simulink model "F16ASYM_Controlled_ACC"  (R2012b)
settings: Solver=ode3  SolverMode=SingleTasking  StartTime=0.0  StopTime=inf  FixedStep=T_sim  RelTol=1e-3
InitFcn:
  | load('NN_c_weights_Last_stable.mat')
values from neighbouring files (symbols this model uses):
  a1 = fitresult.p1    [Stall_protection.m]
  alpha_map_eval = ones(size(M_eval))*NaN    [Auto_trim_aid.m]    (also in Autotrim_maps.mat = [nan nan 0.277598136245 0.119432432992 0.0579479097061 0.027)
  beta_map_eval = ones(size(M_eval))*NaN    [Auto_trim_aid.m]    (also in Autotrim_maps.mat = [nan nan -0.00151549403324 0.00117807579006 -0.0052086799721)
  C_L_0 = fitresult.p2    [Stall_protection.m]
  G_eval = NaN*ones(size(M_sq,2),size(H_sq,2))    [Stall_protection.m]
  H_sq = unique(sort(H_sq))    [Stall_protection.m]
  H_sq_autotrim = min( F_envelope.H_1g):2000:max(F_envelope.H_1g)    [Auto_trim_aid.m]    (also in Autotrim_maps.mat = [0 2000 4000 6000 8000 10000 12000 14000 16000 18000])
  K_b_ACC = params(3)    [Cost_function.m]
  K_b_q = params(4)    [Cost_function.m]
  learning = 20    [Scheduling_desing.m]
  M_sq = unique(sort(M_sq))    [Stall_protection.m]
  M_sq_autotrim = 0:0.1:max(F_envelope.M_1g)    [Auto_trim_aid.m]    (also in Autotrim_maps.mat = [0 0.1 0.2 0.3 0.4 0.5 0.6 0.7 0.8 0.9 1 1.1 ... (21 element)
  Model_used_flag = 1    [Scheduling_desing.m]
  reg_param = 1    [Scheduling_desing.m]
  T_sim = 0.04    [Run_me.m]    (also in Scheduling_desing.m = 0.02)
  tau_ACC = params(1)    [Cost_function.m]
  tau_q = params(2)    [Cost_function.m]
  V_Comp_A_w_z_last = [-0.043311742939 0.0085685727899 -0.0213735657625 0.0330213821126 -0.0306555996667 -0.00573122365227 -0.0106441480787 0.0329440631876 0.0177121952361 -0.0290685435098 -0.0181457235686 -0.0361990502411 ... (1250 elements, 50x25)]    [NN_c_weights_Last_stable.mat]
  V_Comp_last = [-0.0421958473648 0.0184516098779 -0.0436695953504 -0.041154016657 0.00216882652165 -0.0388561228631 0.0327521861474 0.0326079628857 0.0227071838361 -0.0338588476214 0.0161615063846 0.00186003522421 ... (1250 elements, 50x25)]    [NN_c_weights_Last_stable.mat]
  velocity = M_eval(I,J)*a    [Auto_trim_aid.m]    (also in Scheduling_desing.m = M_eval_sche(I,J)*a)
  W_Comp_A_w_z_last = [-0.00689921461652 0.00234704735165 -0.000126421245896 0.00121944724496 6.17702028018e-05 -0.000422762754226 -0.000228913732743 -1.1618795843e-05 7.94007436465e-05 0.000588815786054 2.98617078429e-05 -0.00020420127191 ... (153 elements, 3x51)]    [NN_c_weights_Last_stable.mat]
  W_Comp_last = [-0.00864477030284 0.000183920433695 -0.000300268209456 0.00178165628538 -0.000144806488148 -0.000715209966 -0.000733452792184 5.9552378004e-05 0.000293789747621 0.00184648331608 -0.000150090451416 -0.000741280397229 ... (153 elements, 3x51)]    [NN_c_weights_Last_stable.mat]
undefined symbols (not defined in the file or in its folder): B, DiscIntNeverNeededParam, fi_flag_Simulink, k_B, m_B, sigbuilder_block, Stall_curve, Theta_1_roll_last, Theta_2_roll_last, Theta_3_roll_last, trim_control, trim_state, trim_throttle, V_long_lastA_w_z, V_long_lastAoA, V_roll_last, V_roll_lastMOD, V_yaw_last, W_long_lastA_w_z, W_long_lastAoA, W_roll_last, W_roll_lastMOD, W_yaw_last
libraries: Adaptive_FaultTolerantControl x43, F16_Actuator_Library x14, dspsigops x13, simulink x8, dsparch4 x6, simulink_extras x5, aerolibatmos2 x5, aerolibtransform2 x5, dspmtrx3 x3, qcatlib x2, dspvision x2, dspsnks4 x2
(part 2 of 10)

== system F16ASYM_Controlled_ACC/Cockpit/Joystick ==
  Add1 : Sum
  Add2 : Sum
  Aileron : Selector  InputPortWidth=2  IndexOptions=Index vector (dialog)  Indices=1  OutputSizes=1
  Gain : Gain  Gain=0.01  OutDataTypeStr=double
  Gain{1..2,4,8} (4 alike) : Gain
  Gain3 : Gain  Gain=-1
  Gain5 : Gain  Gain=-10
  Gain6 : Gain  Gain=10  OutDataTypeStr=double
  Gain7 : Gain  Gain=-1
  Integrator Limited2 : Integrator  LimitOutput=on  UpperSaturationLimit=400  LowerSaturationLimit=-400
  Integrator Limited3 : Integrator  LimitOutput=on  UpperSaturationLimit=1  LowerSaturationLimit=-1
  Joystick Input : vrlib/Joystick Input  joyid=1  adjustports=on  forcefeed=off
  Manual Switch : ManualSwitch
  Selector1 : Selector  InputPortWidth=5  IndexOptions=Index vector (dialog)  Indices=1:2  OutputSizes=1
  Selector2 : Selector  InputPortWidth=5  IndexOptions=Index vector (dialog)  Indices=3  OutputSizes=1
  Selector3 : Selector  InputPortWidth=5  IndexOptions=Index vector (dialog)  Indices=4:5  OutputSizes=1
  Selector4 : Selector  InputPortWidth=10  IndexOptions=Index vector (dialog)  Indices=1  OutputSizes=1
  Selector5 : Selector  InputPortWidth=10  IndexOptions=Index vector (dialog)  Indices=4  OutputSizes=1
  Selector6 : Selector  InputPortWidth=10  IndexOptions=Index vector (dialog)  Indices=1  OutputSizes=1
  Selector7 : Selector  InputPortWidth=10  IndexOptions=Index vector (dialog)  Indices=4  OutputSizes=1
  elev : Selector  InputPortWidth=2  IndexOptions=Index vector (dialog)  Indices=2  OutputSizes=1
  speed des : Outport
  Throttle : Outport  Port=2
  Long: Acc : Outport  Port=3
  Roll : Outport  Port=4
  sideslip : Outport  Port=5
  wires:
  Integrator Limited3/1 -> Throttle/1  "Throttle"
  Aileron/1 -> Gain1/1
  Manual Switch/1 -> Aileron/1, elev/1
  Joystick Input/1 -> Selector2/1, Selector3/1, Selector1/1
  Selector1/1 -> Manual Switch/1
  Selector3/1 -> Manual Switch/2
  Selector4/1 -> Gain3/1
  Selector5/1 -> Gain4/1
  Gain3/1 -> Add1/1
  Gain4/1 -> Add1/2
  Add1/1 -> Gain/1
  Gain/1 -> Integrator Limited3/1
  elev/1 -> Gain2/1
  Gain1/1 -> Roll/1
  Selector2/1 -> Gain5/1
  Gain2/1 -> Long: Acc/1
  Gain5/1 -> sideslip/1
  Integrator Limited2/1 -> speed des/1  "Throttle"
  Joystick Input/2 -> Selector5/1, Selector7/1, Selector6/1, Selector4/1
  Selector6/1 -> Gain7/1
  Selector7/1 -> Gain8/1
  Gain7/1 -> Add2/1
  Gain8/1 -> Add2/2
  Add2/1 -> Gain6/1
  Gain6/1 -> Integrator Limited2/1

== system F16ASYM_Controlled_ACC/Cockpit/Signal Builder1 ==
  Demux : Demux  Tag=STV Demux
  FromWs : FromWorkspace  Tag=STV FromWs  VariableName=tuvar  SampleTime=0
      SigBuilderData=|
      | common.afterFinalStr = 'Extrapolate'
      | common.sampleTime = 0
      | dataSet.timeRange = [0 30]
      | dataSet.name = 'Group 1'
      | sbobj.Groups.Name = 'Group 1'
      | sbobj.Groups.Signals(1).Name = 'Signal 1'
      | sbobj.Groups.Signals(1).XData = [0 0.5 0.5 2.5 2.5 30]
      | sbobj.Groups.Signals(1).YData = [0 0 -1 -1 0 0]
      | sbobj.Groups.Signals(2).Name = 'Signal 5'
      | sbobj.Groups.Signals(2).XData = [0 4 4 6 6 30]
      | sbobj.Groups.Signals(2).YData = [0 0 1 1 0 0]
      | sbobj.Groups.Signals(3).Name = 'Signal 6'
      | sbobj.Groups.Signals(3).XData = [0 8 8 10 10 30]
      | sbobj.Groups.Signals(3).YData = [0 0 -0.5 -0.5 0 0]
      | sbobj.Groups.Signals(4).Name = 'Signal 7'
      | sbobj.Groups.Signals(4).XData = [0 12 12 14 14 30]
      | sbobj.Groups.Signals(4).YData = [0 0 0.5 0.5 0 0]
      | sbobj.Groups.TimeRange = [0 30]
  Signal 1 : Outport  Tag=STV Outport
  Signal 5 : Outport  Tag=STV Outport  Port=2
  Signal 6 : Outport  Tag=STV Outport  Port=3
  Signal 7 : Outport  Tag=STV Outport  Port=4
  wires:
  FromWs/1 -> Demux/1
  Demux/1 -> Signal 1/1
  Demux/2 -> Signal 5/1
  Demux/3 -> Signal 6/1
  Demux/4 -> Signal 7/1

== system F16ASYM_Controlled_ACC/Cockpit/Signal Builder2 ==
  Demux : Demux  Tag=STV Demux
  FromWs : FromWorkspace  Tag=STV FromWs  VariableName=tuvar  SampleTime=0
      SigBuilderData=|
      | common.afterFinalStr = 'Extrapolate'
      | common.sampleTime = 0
      | dataSet.timeRange = [0 10]
      | dataSet.name = 'Group 1'
      | sbobj.Groups.Name = 'Group 1'
      | sbobj.Groups.Signals(1).Name = 'Signal 1'
      | sbobj.Groups.Signals(1).XData = [0 5 5 8.02 8.02 10]
      | sbobj.Groups.Signals(1).YData = [0 0 -8.15 -8.15 0.64 0.7]
      | sbobj.Groups.Signals(2).Name = 'Signal 2'
      | sbobj.Groups.Signals(2).XData = [0 10]
      | sbobj.Groups.Signals(2).YData = [0 0]
      | sbobj.Groups.Signals(3).Name = 'Signal 3'
      | sbobj.Groups.Signals(3).XData = [0 10]
      | sbobj.Groups.Signals(3).YData = [0 0]
      | sbobj.Groups.Signals(4).Name = 'Signal 4'
      | sbobj.Groups.Signals(4).XData = [0 10]
      | sbobj.Groups.Signals(4).YData = [0 0]
  Signal 1 : Outport  Tag=STV Outport
  Signal 2 : Outport  Tag=STV Outport  Port=2
  Signal 3 : Outport  Tag=STV Outport  Port=3
  Signal 4 : Outport  Tag=STV Outport  Port=4
  wires:
  FromWs/1 -> Demux/1
  Demux/1 -> Signal 1/1
  Demux/2 -> Signal 2/1
  Demux/3 -> Signal 3/1
  Demux/4 -> Signal 4/1

== matlab function F16ASYM_Controlled_ACC/Primary Controller/P controller + adaptive Isolated NN/On-line (adaptive) multi-layer NNs SIMPL/Roll NN/Roll 1HL NN/Roll NN ==
  data: X_bar input size=[8,1]; v_ad_comp output; e input; P input; B input; Roll_learnign_rate input size=1; Roll_reg_param input size=1; W input size=[1,31]; V input size=[30,8]; v_ad output; Z_norm_unit output; T_sim parameter; W_update output size=[1,31]; V_update output size=[30,8]
function [v_ad_comp,v_ad,Z_norm_unit,W_update,V_update]  = Roll_NN(X_bar,e,P,B,Roll_learnign_rate,Roll_reg_param,W,V,T_sim)

%% Compute prelimiary parametes
zeta= e'*P*B;
s=zeros(30,1);
z=s;
%% Feedforward
z = V*X_bar;
s=sigmoid(V*X_bar);

sigma = [1 ; s ];
% v_ad = W*sigma;

sigma_grad = (sigma.*(ones(size(sigma))-sigma));

%% Compute the gradients or adaptation laws
Gamma_w= Roll_learnign_rate; % W learnign rate
Gamma_v= Roll_learnign_rate; %V learning rate
lambda = Roll_reg_param;

V_dot=zeros(size(V));
W_dot=zeros(size(W'));

W_dot= -Gamma_w*(  (sigma - sigma_grad.*[1;z] ).*zeta  );
W_dot(2:end,1)= W_dot(2:end,1) - Gamma_w*lambda*norm(zeta)*(W(:,2:end))';

M = W'*zeta.*sigma_grad ;
V_dot= -Gamma_v*( M(2:end)*X_bar'  );
V_dot(:,2:end)= V_dot(:,2:end) - Gamma_v*lambda*norm(zeta).*V(:,2:end);


% Other way: Based on notes of Andrew NG
% % % % W_dot=zeros(size(W));
% % % % delta2=W'*zeta.*sigma_grad;
% % % % 
% % % % V_dot = - Gamma_v*( delta2(2:end)*X_bar');
% % % % V_dot(:,2:end)= V_dot(:,2:end) - Gamma_v*lambda*norm(zeta).*V(:,2:end);
% % % % 
% % % % W_dot = - Gamma_w*( zeta*sigma');
% % % % W_dot(:,2:end)= W_dot(:,2:end) - Gamma_w*lambda*norm(zeta)*(W(:,2:end));
% % % % 
% % % % W_dot = W_dot';


%% Adaptation
W_update = W + T_sim*W_dot';
V_update = V + T_sim*V_dot;

%% re-compute v_ad

z = V*X_bar;
s=sigmoid(V*X_bar);

sigma = [1 ; s(:,1) ];
v_ad = W*sigma;

%% Compute v_ad_comp
Z = [ V,zeros(size(V,1),size(W,2));
    zeros(size(W,1),size(V,2)),W];
    
Z_norm = norm(Z,'fro');
Z_max = 2*min(size(W,1),size(W,2) )*min( size(V,1),size(V,2) );
Z_norm_unit = Z_norm;

K_r0= 0;
K_r1= 0;
v_r0 = -K_r0*zeta;
v_r1 = -K_r1*(Z_norm+Z_max)*zeta;
v_ad_comp = v_ad + v_r1 +v_r0;

% % K_r1= 1;
% % v_r1 = - K_r1*(Z_norm+Z_max)*zeta;
% % 
% % v_ad_comp = v_ad + v_r1 ;



end

== matlab function F16ASYM_Controlled_ACC/Anti-windup Calculation/Anti-windup: Reconfigurable/Ang Accel ==
  data: L input; p_dot output; q_dot output; r_dot output; M input; N input; omega_b input
function [p_dot,q_dot,r_dot] = Ang_accel(L,M,N,omega_b)
Jy  = 75673.6;
Jxz = 1331.4; 
Jz  = 85552.1;  
Jx  = 12874.8;
h_E = 216.9;

denom = Jx*Jz - Jxz*Jxz;

% % C1 = ((Jy - Jz)  * Jz  - (Jxz * Jxz))/ Gamma;
% % C2 = ((Jx - Jy + Jz ) * Jxz ) / Gamma;
% % C3 = Jz / Gamma;
% % C4 = Jxz / Gamma;
% % C5 = (Jz - Jx) / Jy;
% % C6 = Jxz / Jy ;
% % C7 = 1 / Jy;
% % C8 = (Jx * (Jx - Jy ) + Jxz * Jxz) / Gamma;
% % C9 = Jx / Gamma;


p_dot =  (Jz*L + Jxz*N - (Jz*(Jz-Jy)+Jxz*Jxz)*omega_b(2)*omega_b(3) + Jxz*(Jx-Jy+Jz)*omega_b(1)*omega_b(2) + Jxz*omega_b(2)*h_E)/denom;

q_dot = (M + (Jz-Jx)*omega_b(1)*omega_b(3) - Jxz*(omega_b(1)*omega_b(1)-omega_b(3)*omega_b(3)) - omega_b(3)*h_E)/Jy;


r_dot = (Jx*N + Jxz*L + (Jx*(Jx-Jy)+Jxz*Jxz)*omega_b(1)*omega_b(2) - Jxz*(Jx-Jy+Jz)*omega_b(2)*omega_b(3) +  Jx*omega_b(2)*h_E)/denom;

== matlab function F16ASYM_Controlled_ACC/Anti-windup Calculation/Anti-windup: NO reconfigurable/Antiwindup calculation ==
  data: Ang_acell_comm input; AWU output; Ang_acell_achieved input; Saturations input; B input; deflections input
function AWU = AWU_calculation(Ang_acell_comm,Ang_acell_achieved,Saturations,B,deflections)
% Computing Saturation limits
sup_limit = [24,24,21,21,29,25,25]-1;
inf_limit = [-24,-24,-21,-21,-29,0,0]+1;

for i=1:7
    Saturations(i) = Saturation_smooth(abs(Saturations(i)),deflections(i),sup_limit(i),inf_limit(i));
end
Sat_B = B*Saturations;
B_max = B*ones(7,1);

AWU=zeros(3,1);

%% Method A
% % psi = 0.01; % % of the effort above the one we consider manouvreability is reduced
% % for i=1:3
% %     if i==1 && sign(deflections(3))== sign(deflections(4)) && abs(Sat_B(i))>psi*abs(B_max(i))
% %         AWU(2) = Ang_acell_comm(2) - Ang_acell_achieved(2); % we have to desaturate longitudinally not laterally
% %     elseif  i==1 && sign(deflections(3))~= sign(deflections(4)) && abs(Sat_B(i))>psi*abs(B_max(i))
% %         AWU(i) = Ang_acell_comm(i) - Ang_acell_achieved(i);
% %     elseif i~=1 && abs(Sat_B(i))>psi*abs(B_max(i))
% %         AWU(i) = Ang_acell_comm(i) - Ang_acell_achieved(i);
% %     end 
% % end

%% Method B
% % % % Long
% % % if Saturations(1)~=0 || Saturations(2)~=0 ||  Saturations(6)~=0 || Saturations(7)~=0 || ((Saturations(3)~=0 || Saturations(4)~=0) && sign(deflections(3))== sign(deflections(4)) ) 
% % %     AWU(2) = Ang_acell_comm(2) - Ang_acell_achieved(2);
% % % end
% % % % Lat-dir
% % % if ((Saturations(3)~=0 || Saturations(4)~=0) && sign(deflections(3)) ~= sign(deflections(4)) )  || Saturations(5)~=0 || Saturations(6)~=0 || Saturations(7)~=0
% % %     AWU(1) = Ang_acell_comm(1) - Ang_acell_achieved(1);
% % %     AWU(3) = Ang_acell_comm(3) - Ang_acell_achieved(3);
% % % 
% % % end



%% Method C
for i=1:3
        AWU(i) = (Ang_acell_comm(i) - Ang_acell_achieved(i))*Sat_B(i)/norm(B(i,:));
end

end

function Saturation_out = Saturation_smooth(Saturation,angle,sup_limit,inf_limit)

a=5;
Saturation_out  = ( 1 - 1./(1+exp(-a*(angle-inf_limit ))) + 1./(1+exp(-a*(angle-sup_limit ))) )*Saturation;


end

== matlab function F16ASYM_Controlled_ACC/Primary Controller/P controller + adaptive Crossed NN + AWU+Lim /Longitudinal Controller: AoA or A_w_z/Longitudinal controller in A_w_z/Stall protection/MATLAB Function ==
  data: alpha_dot input; alpha_dot_out output; alpha input
function alpha_dot_out = AoA_limit(alpha_dot,alpha)
a=180/pi;
AoA_sup = deg2rad(18);
AoA_inf = -deg2rad(18);


if (alpha>0 & alpha_dot<0)  || (alpha<0 & alpha_dot>0) 
    alpha_dot_out = alpha_dot;
else
    alpha_dot_out  = ( 2./(1+exp(-a*(alpha-AoA_inf ))) -1 -2./(1+exp(-a*(alpha-AoA_sup ))) )*alpha_dot;
end

== matlab function F16ASYM_Controlled_ACC/Primary Controller/P  + Crossed NN + AWU+Lim + hand-over/P controller + adaptive Crossed NN + AWU+Lim    in ACC /Complete crossed On-line (adaptive) multi-layer NN: A_w_z/Cross NN A_w_z ==
  data: X_bar input size=[25,1]; v_ad_comp output; e input; Factor_F input; K_roll input; Ks_long input; Ks_yaw input; B input; Learnign_rate input size=1; Reg_param input size=1; AWU input; W input size=[3,51]; V input size=[50,25]; v_ad output; Z_norm_unit output; T_sim parameter; W_update output; V_update output
function [v_ad_comp,v_ad,Z_norm_unit,W_update,V_update]  = Cross_NN(X_bar,e,Factor_F, K_roll,Ks_long,Ks_yaw,B,Learnign_rate,Reg_param,AWU,W,V,T_sim)

%% Compute prelimiary parametes
% Compute P with regular Lyapunov equation solution
P_roll=1/K_roll;
P_long =  [   1/Ks_long(1) , Factor_F/(Ks_long(1)^2+Ks_long(1)*Ks_long(2));
     1/(Ks_long(1)^2+Ks_long(1)*Ks_long(2)) ,(Ks_long(1)^2+Ks_long(1)*Ks_long(2)+Factor_F^2)/(Ks_long(2)^2*Ks_long(1)+Ks_long(2)*Ks_long(1)^2) ];
P_yaw = [   1/Ks_yaw(1) , 1/(Ks_yaw(1)^2+Ks_yaw(1)*Ks_yaw(2));
     1/(Ks_yaw(1)^2+Ks_yaw(1)*Ks_yaw(2)) ,(Ks_yaw(1)^2+Ks_yaw(1)*Ks_yaw(2)+1)/(Ks_yaw(2)^2*Ks_yaw(1)+Ks_yaw(2)*Ks_yaw(1)^2) ];
 
P = blkdiag(P_roll,P_long,P_yaw);

% % % % Compute P with on-line Lyapunov equation solution
% % % CROSS = 0;
% % % A = [ -K_roll,0,CROSS,0,0;0,-Ks_long(1),1,0,0;
% % %     0,0,-Ks_long(2),0,0;0,0,0,-Ks_yaw(1),Factor_F;0,0,0,0,-Ks_yaw(2)];
% % % 
% % % coder.extrinsic('lyap')
% % % P = A;
% % % P = lyap(A,2*diag(ones(5,1)));



K_awu = 1.2;
zeta= e'*P*B;


% Introduce Anti-windup
zeta = zeta - K_awu*AWU'.*T_sim; 

% Convergence limitation
if norm(zeta)>2/(T_sim*Learnign_rate*Reg_param)
    zeta = (zeta./norm(zeta)).*(1.8/(T_sim*Learnign_rate*Reg_param));
end

%% Feedforward
z = V*X_bar;
s=sigmoid(V*X_bar);

sigma = [1 ; s ];
% v_ad = W*sigma;

sigma_grad = (sigma.*(ones(size(sigma))-sigma));

%% Compute the gradients or adaptation laws
Gamma_w= Learnign_rate; % W learnign rate
Gamma_v= Learnign_rate; %V learning rate
lambda = Reg_param;

V_dot=zeros(size(V));
W_dot=zeros(size(W));

W_dot= -Gamma_w*(  (sigma - sigma_grad.*[1;z] )*zeta  )';
W_dot(:,2:end)= W_dot(:,2:end) - Gamma_w*lambda*norm(zeta)*(W(:,2:end));

M = W'*zeta'.*sigma_grad ;
V_dot= -Gamma_v*( M(2:end)*X_bar'  );
V_dot(:,2:end)= V_dot(:,2:end) - Gamma_v*lambda*norm(zeta).*V(:,2:end);

% % % Other way: Based on notes of Andrew NG
% % 
% % delta2=W'*zeta'.*sigma_grad;
% % 
% % V_dot = - Gamma_v*( delta2(2:end)*X_bar');
% % V_dot(:,2:end)= V_dot(:,2:end) - Gamma_v*lambda*norm(zeta).*V(:,2:end);
% % 
% % W_dot = - Gamma_w*( sigma*zeta)';
% % W_dot(:,2:end)= W_dot(:,2:end) - Gamma_w*lambda*norm(zeta)*(W(:,2:end));



%% Adaptation
W_update = W + T_sim*W_dot;
V_update = V + T_sim*V_dot;
% 
%% Re-compute v_ad

s=sigmoid(V_update*X_bar);

sigma = [1 ; s(:,1) ];
v_ad = W_update*sigma;

%% Compute v_ad_comp
Z = [ V,zeros(size(V,1),size(W,2));
    zeros(size(W,1),size(V,2)),W];
    
Z_norm = norm(Z,'fro');
Z_max = 2*min(size(W,1),size(W,2) )*min( size(V,1),size(V,2) );
Z_norm_unit = Z_norm;

K_r0= 0;
K_r1= 0;
v_r0 = -K_r0*zeta';
v_r1 = -K_r1*(Z_norm+Z_max)*zeta';

v_ad_comp = v_ad + v_r1 +v_r0;

% % % Normalization of matrices
% % if Z_norm>Z_max
% %     V = (V.*Z_max)./Z_norm;
% %     W = (W.*Z_max)./Z_norm;
% % end
end

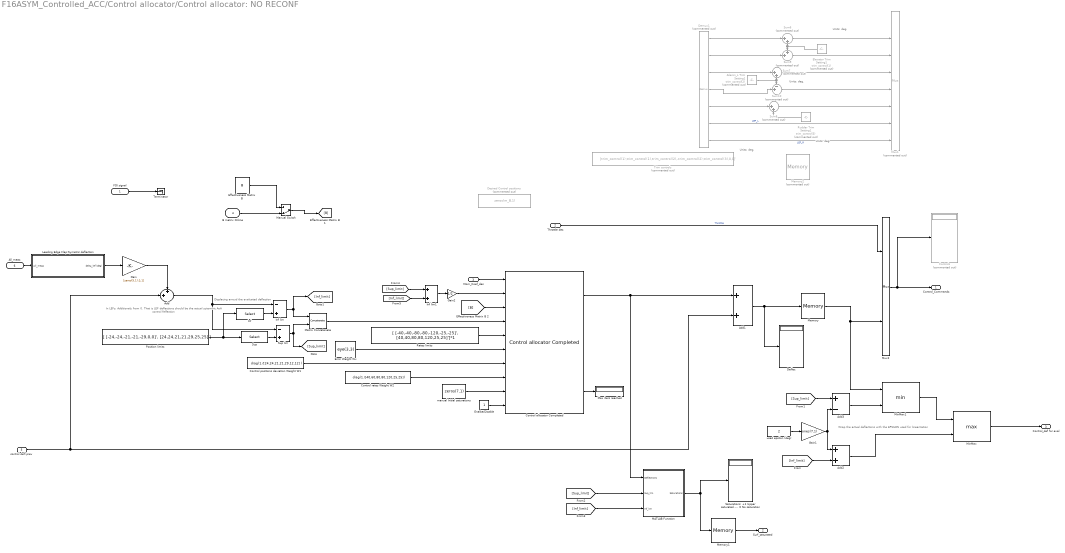
== system F16ASYM_Controlled_ACC/Control allocator/Control allocator: NO RECONF ==
  note: Wrap the actual deflections with the EPSILON
      |  used for linearization
  note: Units: deg.
  note: Units: deg.
  note: Units: deg.
  note: Units: deg.
  note: In LEFs: Additionaly from 0.  That is LEF deflections should be
      | the actual sytemtric AoA control felfection
  note: Displacing arroud the evaluated deflection
  FDI signal : Inport
  Throttle des : Inport  Port=2
  Mom_Coef_des : Inport  Port=3
  B matrix Online : Inport  Port=4
  control defl prev : Inport  Port=5
  All_meas : Inport  Port=6
  Add : Sum  Inputs=++|
  Add1 : Sum
  Add2 : Sum
  Add3 : Sum  Inputs=+-
  Aileron_L Trim Setting1 : Constant  Commented=on  Value=trim_control(2)
  "Control allocator Completed " : qcatlib/Control allocator Completed   alg=SLS  CA_type=QP  iter_max=100  gamma=1e6  k_B=3  m_B=7  T=T_sim  tol=1e-5
  Control positions deviation Weight W1 : Constant  Value=diag(1./[24,24,21,21,29,12,12] )
  Control rates Weight W2 : Constant  Value=diag(1./[40,60,80,80,120,25,25])
  Controls : Display  Commented=on
  Deflec : Display
  Demux1 : Demux  Commented=on  Outputs=[1,1,1,1,1,1,1]
  Desired Control positions : Constant  Commented=on  Value=zeros(m_B,1)
  Effectiveness Matrix B : Constant  Value=B
  Elevator Trim Setting1 : Constant  Commented=on  Value=trim_control(1)  VectorParams1D=off
  Enalbe/Disable : Constant
  Error Weight Wv : Constant  Value=eye(3,3)
  Gain : Gain  Gain=[zeros(5,1);1;1]
  Gain1 : Gain  Gain=ones(7,1)
  Gain2 : Gain  Gain=1/2
  Inf : Selector  NumberOfDimensions=2  InputPortWidth=3  IndexOptions=Index vector (dialog),Index vector (dialog)  Indices=[1:7],1  OutputSizes=1,1
  Inf lim : Sum  Inputs=-+
  Inf lim1 : Sum
  Leading Edge Flap:Symetric deflection : Subsystem
  MATLAB Function : MATLAB Function  TreatAsAtomicUnit=on
  Manual Switch : ManualSwitch  CurrentSetting=0
  Matrix Concatenate : Concatenate  Mode=Multidimensional array  ConcatenateDimension=2
  Max iters reached : Display
  Memory : Memory  X0=[trim_control(1),trim_control(1),trim_control(2),-trim_control(2),trim_control(3),0,0]'
  Memory1 : Memory  X0=zeros(7,1)
  Memory2 : Memory  Commented=on  X0=zeros(7,1)
  MinMax : MinMax  Function=max  Inputs=2
  MinMax1 : MinMax  Inputs=2
  Mux1 : Mux  Commented=on  Inputs=8
  Mux2 : Mux  Inputs=[1 7]
  Position limits : Constant  Value=[ [-24,-24,-21,-21,-29,0,0]', [24,24,21,21,29,25,25]']
  Rates limits : Constant  Value=[ [-40,-40,-80,-80,-120,-25,-25]', [40,40,80,80,120,25,25]']*1
  Rudder Trim Setting1 : Constant  Commented=on  Value=trim_control(3)
  Saturations: +1 Upper saturated -1 Lower saturated 0 No saturation : Display
  Sum10 : Sum  Commented=on  Inputs=-+|  SaturateOnIntegerOverflow=on  InputSameDT=on  OutDataTypeStr=Inherit: Same as first input
  Sum6 : Sum  Commented=on  Inputs=|++  SaturateOnIntegerOverflow=on  InputSameDT=on  OutDataTypeStr=Inherit: Same as first input
  Sum7 : Sum  Commented=on  Inputs=|++  SaturateOnIntegerOverflow=on  InputSameDT=on  OutDataTypeStr=Inherit: Same as first input
  Sum8 : Sum  Commented=on  Inputs=|++  SaturateOnIntegerOverflow=on  InputSameDT=on  OutDataTypeStr=Inherit: Same as first input
  Sum9 : Sum  Commented=on  Inputs=++|  SaturateOnIntegerOverflow=on  InputSameDT=on  OutDataTypeStr=Inherit: Same as first input
  Sup : Selector  NumberOfDimensions=2  InputPortWidth=3  IndexOptions=Index vector (dialog),Index vector (dialog)  Indices=[1:7],2  OutputSizes=1,1
  Sup lim : Sum  Inputs=-+
  Terminator : Terminator
  "Trim controls " : Constant  Commented=on  Value=[trim_control(1),trim_control(1),trim_control(2),-trim_control(2),trim_control(3),0,0]'
  manual Initial saturations : Constant  Value=zeros(7,1)
  used epsilon (deg) : Constant  Value=2
  Control_Commands : Outport
  Surf_saturated : Outport  Port=2
  Control_def for eval : Outport  Port=3
  wires:
  MinMax/1 -> Control_def for eval/1
  MinMax1/1 -> MinMax/1
  Add3/1 -> MinMax1/2
  used epsilon (deg)/1 -> Gain1/1
  [Inf_limit] -> Add2/2
  Gain1/1 -> Add3/2, Add2/1
  [Sup_limit] -> Add3/1
  Add2/1 -> MinMax/2
  Memory/1 -> Mux2/2, MinMax1/1
  Add1/1 -> Memory/1, Deflec/1
  Demux1/5 -> Sum8/1
  Rudder Trim Setting1/1 -> Sum8/2
  Elevator Trim Setting1/1 -> Sum9/1, Sum6/2
  Demux1/4 -> Sum10/2
  Demux1/3 -> Sum7/1
  Demux1/2 -> Sum9/2
  Demux1/1 -> Sum6/1
  Demux1/7 -> Mux1/8  "LEF_R"
  Demux1/6 -> Mux1/7  "LEF_L"
  Sum9/1 -> Mux1/3
  Sum6/1 -> Mux1/2
  Aileron_L Trim Setting1/1 -> Sum10/1, Sum7/2
  Sum10/1 -> Mux1/5
  Sum8/1 -> Mux1/6
  Sum7/1 -> Mux1/4
  ? -> Mux1/1  "Throttle"
  Control positions deviation Weight W1/1 -> "Control allocator Completed "/7
  FDI signal/1 -> Terminator/1
  Leading Edge Flap:Symetric deflection/1(delta_lef (deg)) -> Gain/1
  All_meas/1 -> Leading Edge Flap:Symetric deflection/1(All_meas)
  Gain/1 -> Add/1
  control defl prev/1 -> Add1/2, Add/2
  Manual Switch/1 -> [B]
  Effectiveness Matrix B/1 -> Manual Switch/1
  B matrix Online/1 -> Manual Switch/2
  "Control allocator Completed "/1 -> MATLAB Function/1(Deflections), Add1/1
  Enalbe/Disable/1 -> "Control allocator Completed "/10
  manual Initial saturations/1 -> "Control allocator Completed "/9
  "Control allocator Completed "/3 -> Max iters reached/1
  [B] -> "Control allocator Completed "/3
  Sup lim/1 -> [Sup_limit], Matrix Concatenate/2
  Inf lim/1 -> [Inf_limit], Matrix Concatenate/1
  Matrix Concatenate/1 -> "Control allocator Completed "/4
  Inf/1 -> Inf lim/2
  Add/1 -> Inf lim/1, Sup lim/1
  Sup/1 -> Sup lim/2
  Control rates Weight W2/1 -> "Control allocator Completed "/8
  Error Weight Wv/1 -> "Control allocator Completed "/6
  Rates limits/1 -> "Control allocator Completed "/5
  Position limits/1 -> Sup/1, Inf/1
  Gain2/1 -> "Control allocator Completed "/2
  Mux2/1 -> Control_Commands/1, Controls/1
  Throttle des/1 -> Mux2/1  "Throttle"
  Mom_Coef_des/1 -> "Control allocator Completed "/1
  [Sup_limit] -> MATLAB Function/2(Sup_lim)
  [Inf_limit] -> MATLAB Function/3(Inf_lim)
  MATLAB Function/1(Saturations) -> Memory1/1, Saturations: +1 Upper saturated -1 Lower saturated 0 No saturation/1
  [Sup_limit] -> Inf lim1/1
  [Inf_limit] -> Inf lim1/2
  Inf lim1/1 -> Gain2/1
  Memory1/1 -> Surf_saturated/1

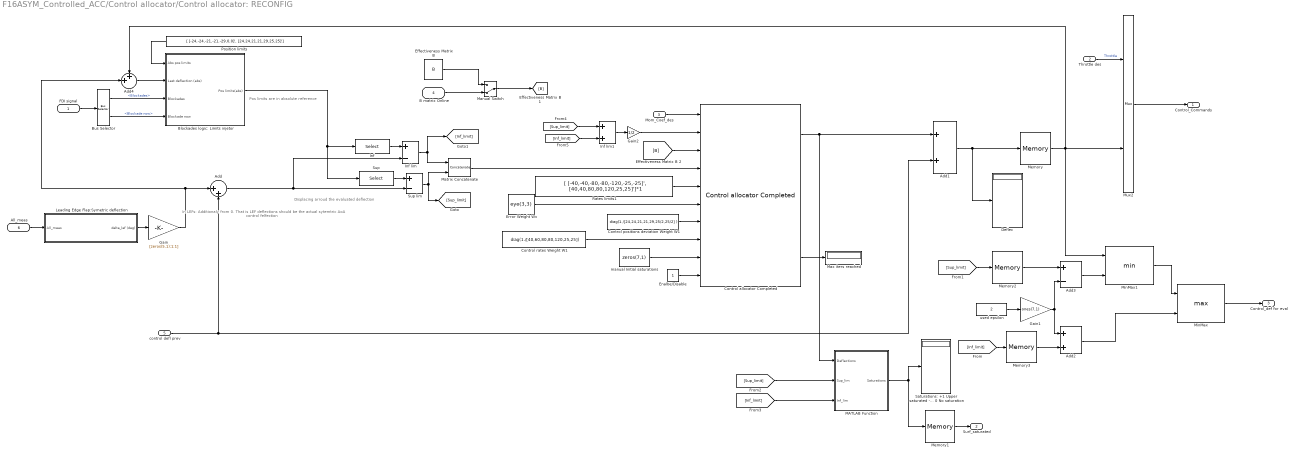
== system F16ASYM_Controlled_ACC/Control allocator/Control allocator: RECONFIG ==
  note: Pos limits are in absolute reference
  note: In LEFs: Additionaly from 0.  That is LEF deflections should be
      | the actual sytemtric AoA control felfection
  note: Displacing arroud the evaluated deflection
  FDI signal : Inport
  Throttle des : Inport  Port=2
  Mom_Coef_des : Inport  Port=3
  B matrix Online : Inport  Port=4
  control defl prev : Inport  Port=5
  All_meas : Inport  Port=6
  Add : Sum  Inputs=|++
  Add1 : Sum
  Add2 : Sum
  Add3 : Sum  Inputs=+-
  Add4 : Sum  Inputs=++|
  Blockades logic: Limits injetor : Subsystem
  Bus Selector : BusSelector  OutputSignals=Blockades,Blockade now
  "Control allocator Completed " : qcatlib/Control allocator Completed   alg=WLS  CA_type=QP  iter_max=100  gamma=1e8  k_B=3  m_B=7  T=T_sim  tol=1e-5
  Control positions deviation Weight W1 : Constant  Value=diag(1./[24,24,21,21,29,25/2,25/2] )
  Control rates Weight W1 : Constant  Value=diag(1./[40,60,80,80,120,25,25])
  Deflec : Display
  Effectiveness Matrix B : Constant  Value=B
  Enalbe/Disable : Constant
  Error Weight Wv : Constant  Value=eye(3,3)
  Gain : Gain  Gain=[zeros(5,1);1;1]
  Gain1 : Gain  Gain=ones(7,1)
  Gain2 : Gain  Gain=1/2
  Inf : Selector  NumberOfDimensions=2  InputPortWidth=3  IndexOptions=Index vector (dialog),Index vector (dialog)  Indices=[1:7],1  OutputSizes=1,1
  Inf lim : Sum  Inputs=+-
  Inf lim1 : Sum
  Leading Edge Flap:Symetric deflection : Subsystem
  MATLAB Function : MATLAB Function  TreatAsAtomicUnit=on
  Manual Switch : ManualSwitch  CurrentSetting=0
  Matrix Concatenate : Concatenate  Mode=Multidimensional array  ConcatenateDimension=2
  Max iters reached : Display
  Memory : Memory  X0=[trim_control(1),trim_control(1),trim_control(2),-trim_control(2),trim_control(3),0,0]'
  Memory1 : Memory  X0=zeros(7,1)
  Memory2 : Memory  X0=[24,24,21,21,29,25,25]'
  Memory3 : Memory  X0=[-24,-24,-21,-21,-29,0,0]'
  MinMax : MinMax  Function=max  Inputs=2
  MinMax1 : MinMax  Inputs=2
  Mux2 : Mux  Inputs=[1 7]
  Position limits : Constant  Value=[ [-24,-24,-21,-21,-29,0,0]', [24,24,21,21,29,25,25]']
  Rates limits1 : Constant  Value=[ [-40,-40,-80,-80,-120,-25,-25]', [40,40,80,80,120,25,25]']*1
  Saturations: +1 Upper saturated -1 Lower saturated 0 No saturation : Display
  Sup : Selector  NumberOfDimensions=2  InputPortWidth=3  IndexOptions=Index vector (dialog),Index vector (dialog)  Indices=[1:7],2  OutputSizes=1,1
  Sup lim : Sum  Inputs=+-
  manual Initial saturations : Constant  Value=zeros(7,1)
  used epsilon : Constant  Value=2
  Control_Commands : Outport
  Surf_saturated : Outport  Port=2
  Control_def for eval : Outport  Port=3
  wires:
  Mom_Coef_des/1 -> "Control allocator Completed "/1
  Throttle des/1 -> Mux2/1  "Throttle"
  Mux2/1 -> Control_Commands/1
  Rates limits1/1 -> "Control allocator Completed "/5
  Error Weight Wv/1 -> "Control allocator Completed "/6
  Control rates Weight W1/1 -> "Control allocator Completed "/8
  Sup/1 -> Sup lim/1
  Add/1 -> Inf lim/2, Sup lim/2
  Inf/1 -> Inf lim/1
  Matrix Concatenate/1 -> "Control allocator Completed "/4
  Inf lim/1 -> Matrix Concatenate/1, [Inf_limit]
  Sup lim/1 -> Matrix Concatenate/2, [Sup_limit]
  [B] -> "Control allocator Completed "/3
  "Control allocator Completed "/3 -> Max iters reached/1
  manual Initial saturations/1 -> "Control allocator Completed "/9
  Enalbe/Disable/1 -> "Control allocator Completed "/10
  B matrix Online/1 -> Manual Switch/2
  Effectiveness Matrix B/1 -> Manual Switch/1
  control defl prev/1 -> Add1/2, Add/2
  Gain/1 -> Add/1, Add4/2
  All_meas/1 -> Leading Edge Flap:Symetric deflection/1(All_meas)
  Leading Edge Flap:Symetric deflection/1(delta_lef (deg)) -> Gain/1
  Control positions deviation Weight W1/1 -> "Control allocator Completed "/7
  Add1/1 -> Deflec/1, Memory/1
  Memory/1 -> MinMax1/1, Mux2/2, Add4/1
  Add2/1 -> MinMax/2
  [Sup_limit] -> Memory2/1
  Gain1/1 -> Add2/1, Add3/2
  [Inf_limit] -> Memory3/1
  used epsilon/1 -> Gain1/1
  Add3/1 -> MinMax1/2
  MinMax1/1 -> MinMax/1
  MinMax/1 -> Control_def for eval/1
  Blockades logic: Limits injetor/1(Pos limits(abs)) -> Inf/1, Sup/1
  Bus Selector/1 -> Blockades logic: Limits injetor/3(Blockades)  "<Blockades>"
  Bus Selector/2 -> Blockades logic: Limits injetor/4(Blockade now)  "<Blockade now>"
  FDI signal/1 -> Bus Selector/1
  Add4/1 -> Blockades logic: Limits injetor/2(Last deflection (abs))
  Position limits/1 -> Blockades logic: Limits injetor/1(Abs pos limits)
  Manual Switch/1 -> [B]
  [Sup_limit] -> Inf lim1/1
  [Inf_limit] -> Inf lim1/2
  Inf lim1/1 -> Gain2/1
  Gain2/1 -> "Control allocator Completed "/2
  "Control allocator Completed "/1 -> Add1/1, MATLAB Function/1(Deflections)
  [Sup_limit] -> MATLAB Function/2(Sup_lim)
  [Inf_limit] -> MATLAB Function/3(Inf_lim)
  MATLAB Function/1(Saturations) -> Memory1/1, Saturations: +1 Upper saturated -1 Lower saturated 0 No saturation/1
  Memory1/1 -> Surf_saturated/1
  Memory2/1 -> Add3/1
  Memory3/1 -> Add2/2

== system F16ASYM_Controlled_ACC/Environment params Estimations/Mach number ==
  V : Inport
  a : Inport  Port=2
  Product1 : Product  Inputs=*/  SaturateOnIntegerOverflow=on  InputSameDT=on  OutDataTypeStr=Inherit: Same as first input
  Mach : Outport
  wires:
  Product1/1 -> Mach/1
  V/1 -> Product1/1
  a/1 -> Product1/2

== system F16ASYM_Controlled_ACC/F-16 Non-linear Plant/SYM and ASYM model: No reconfigurable ==
  note: Mdoel used  Flage tells the plant
      |  if Asymetric or symetric model is used:
      | 0: Symetric Model
      | 1: Asymetric model
  note: INPUTS
      | States:
      | 1. North Position
      | 2. East position
      | 3. Altitude
      | 4. Phi
      | 5. Theta
      | 6. Psi
      | 7. Total velocity
      | 8. alpha in rad
      | 9. beta in rads
      | 10. P
      | 11. Q
      | 12. R
      | 13. POW
      |
      | Controls:
      | 14. Throttle
      | 15. Elevator_L in deg
      | 16. Elevator_R in deg
      | 17. Aileron_L
      | 18. Aileron_R
      | 19. Rudder
      | 20. LEF_L
      | 21. LEF_R
      |
      | 22. Fidelity Flag
      |
      | 23. Model used: Asymetric or Symetric
  note: Fidelity Flage tells nlplant
      | which Model to use:
      | 0: Low Fidelity
      | 1: High Fidelity
  note: OUTPUTS
      | States:
      | 1. DEV North Position
      | 2. DEV East position
      | 3. DEV Altitude
      | 4.DEV  Phi
      | 5. DEV Theta
      | 6. DEV Psi
      | 7. DEV Total velocity
      | 8.DEV alpha in rad
      | 9.DEV  beta in rads
      | 10. DEV P
      | 11. DEV Q
      | 12. DEV R
      | 13. DEV POW
      |
      | Other outputs:
      | Accels of CG:
      | 14. anx_cg
      | 15. any_cg
      | 16. anz_cg
      | 17. mach
      | 18. qbar
      | 19. ps   Static Pressure
  note: Add the sytmetric deflection of the LEFs
  States : Inport
  Reconf params : Inport  Port=2
  Control Comands : Inport  Port=3
  Acels actual : Scope
      settings: YMin=-0.04  YMax=0.09  SaveName=ScopeData14
  Actuators Dynamcis : Subsystem  TreatAsAtomicUnit=on
  Bus Creator : BusCreator  Inputs=12
  Bus Creator1 : BusCreator  Inputs=2
  Demux : Demux  Outputs=[13 6]
  Demux1 : Demux  Outputs=8
  F16 nlsim nlplant Asymetrical : MATLABFcn  MATLABFcn=nlplantASYM  OutputDimensions=19  OutputSignalType=real
  Fidelity Flag : Constant  Value=fi_flag_Simulink
  Integrate F16 State Derivatives : Integrator  InitialCondition=trim_state
  Leading Edge Flap:Symetric deflection : Subsystem
  Model used flag : Constant  Value=Model_used_flag
  Mux1 : Mux  Inputs=8
  Mux5 : Mux  Inputs=[13 8 1 1]
  Rotation Angles to Direction Cosine Matrix : aerolibtransform2/Rotation Angles to Direction Cosine Matrix  rotationOrder=ZYX
  Selector : Selector  InputPortWidth=13  IndexOptions=Index vector (dialog)  Indices=[1:3]  OutputSizes=1
  Selector1 : Selector  InputPortWidth=13  IndexOptions=Index vector (dialog)  Indices=[1:3]  OutputSizes=1
  Selector2 : Selector  InputPortWidth=13  IndexOptions=Index vector (dialog)  Indices=[7]  OutputSizes=1
  Selector3 : Selector  InputPortWidth=13  IndexOptions=Index vector (dialog)  Indices=[8:9]  OutputSizes=1
  Selector4 : Selector  InputPortWidth=13  IndexOptions=Index vector (dialog)  Indices=[10:12]  OutputSizes=1
  Selector5 : Selector  InputPortWidth=13  IndexOptions=Index vector (dialog)  Indices=[4:6]  OutputSizes=1
  Selector6 : Selector  InputPortWidth=6  IndexOptions=Index vector (dialog)  Indices=[1:3]  OutputSizes=1
  Selector7 : Selector  InputPortWidth=3  IndexOptions=Index vector (dialog)  Indices=[3 2 1]  OutputSizes=1
  Selector9 : Selector  InputPortWidth=13  IndexOptions=Index vector (dialog)  Indices=[10:12]  OutputSizes=1
  Sum1 : Sum  Inputs=|++  SaturateOnIntegerOverflow=on  InputSameDT=on  OutDataTypeStr=Inherit: Same as first input
  Sum9 : Sum  Inputs=|++  SaturateOnIntegerOverflow=on  InputSameDT=on  OutDataTypeStr=Inherit: Same as first input
  Output_bus : Outport
  Actual control def : Outport  Port=2
  wires:
  Selector7/1 -> Rotation Angles to Direction Cosine Matrix/1
  Demux/2 -> Bus Creator/3, Selector6/1  "Other outs"
  Selector6/1 -> Bus Creator/11  "an_b_CG"
  Selector5/1 -> Bus Creator/9, Selector7/1  "euler"
  Selector4/1 -> Bus Creator/8  "p,q,r"
  Selector3/1 -> Bus Creator/7  "alpha,beta"
  Selector2/1 -> Bus Creator/6  "TAS"
  Selector1/1 -> Bus Creator/5  "V_e"
  Selector/1 -> Bus Creator/4  "X_e"
  Demux/1 -> Integrate F16 State Derivatives/1, Selector1/1, Bus Creator/1, Selector9/1  "States_dot_out"
  Actuators Dynamcis/3(Throttle_meas) -> Bus Creator/12  "Throttle"
  Selector9/1 -> Acels actual/1
  Mux1/1 -> Actuators Dynamcis/1(Control_commands)
  Sum1/1 -> Mux1/8
  Sum9/1 -> Mux1/7
  Demux1/6 -> Mux1/6
  Demux1/4 -> Mux1/4
  Demux1/2 -> Mux1/2
  Demux1/1 -> Mux1/1
  Demux1/3 -> Mux1/3
  Demux1/5 -> Mux1/5
  Demux1/7 -> Sum9/1
  Demux1/8 -> Sum1/1
  Model used flag/1 -> Mux5/4
  F16 nlsim nlplant Asymetrical/1 -> Demux/1  "OUTPUTS"
  Mux5/1 -> F16 nlsim nlplant Asymetrical/1  "INPUTS"
  States/1 -> Mux5/1
  Control Comands/1 -> Demux1/1
  Fidelity Flag/1 -> Mux5/3
  Bus Creator/1 -> Leading Edge Flap:Symetric deflection/1(state), Output_bus/1
  Rotation Angles to Direction Cosine Matrix/1 -> Bus Creator/10  "DCM_b"
  Integrate F16 State Derivatives/1 -> Bus Creator/2, Selector/1, Selector2/1, Selector3/1, Selector4/1, Selector5/1  "States_out"
  Actuators Dynamcis/2(Dec_Control_def) -> Mux5/2
  Leading Edge Flap:Symetric deflection/1(delta_lef (deg)) -> Bus Creator1/1, Sum1/2, Sum9/2  "Symetric_LEF_defl"
  Bus Creator1/1 -> Actual control def/1
  Actuators Dynamcis/1(Control Defl Plot) -> Bus Creator1/2  "actual_control_defl"

== system F16ASYM_Controlled_ACC/F-16 Non-linear Plant/SYM and ASYM model: RECONFIGURABLE ==
  note: Add the sytmetric
      |  deflection of the LEFs
  note: OUTPUTS
      | States:
      | 1. DEV North Position
      | 2. DEV East position
      | 3. DEV Altitude
      | 4.DEV  Phi
      | 5. DEV Theta
      | 6. DEV Psi
      | 7. DEV Total velocity
      | 8.DEV alpha in rad
      | 9.DEV  beta in rads
      | 10. DEV P
      | 11. DEV Q
      | 12. DEV R
      | 13. DEV POW
      |
      | Other outputs:
      | Accels of CG:
      | 14. anx_cg
      | 15. any_cg
      | 16. anz_cg
      | 17. mach
      | 18. qbar
      | 19. ps   Static Pressure
  note: Fidelity Flage tells nlplant
      | which Model to use:
      | 0: Low Fidelity
      | 1: High Fidelity
  note: INPUTS
      | States:
      | 1. North Position
      | 2. East position
      | 3. Altitude
      | 4. Phi
      | 5. Theta
      | 6. Psi
      | 7. Total velocity
      | 8. alpha in rad
      | 9. beta in rads
      | 10. P
      | 11. Q
      | 12. R
      | 13. POW
      |
      | Controls:
      |
      | 14. Throttle
      | 15. Elevator_L in deg
      | 16. Elevator_R in deg
      | 17. Aileron_L
      | 18. Aileron_R
      | 19. Rudder
      | 20. LEF_L
      | 21. LEF_R
      |
      | 22. Fidelity Flag
      |
      | 23. Model used: Asymetric or Symetric
      |
      | RECONFIGURATION PARAMETERS
      |
      | 24. mass  Estimated mass
      | 25. S_current_L
      | 26. S_current_R
      | 27. S_fin_current
      | 28. x_cg
      | 29. Jy
      | 30. Jxz
      | 31. Jz
      | 32. Jx
      | 33. EFF_el_L
      | 34. EFF_el_R
      | 35. EFF_ail_L
      | 36. EFF_ail_R
      | 37. EFF_rud
      | 38. EFF_lef_L
      | 39. EFF_lef_R
      | 40. Delta_C_Lift_X
      | 41. Delta_C_Drag_X
      | 42. Delta_C_m_X
  note: Mdoel used  Flage tells the plant
      |  if Asymetric or symetric model is used:
      | 0: Symetric Model
      | 1: Asymetric model
  States : Inport
  Reconf params : Inport  Port=2
  Control Comands : Inport  Port=3
  Acels actual : Scope
      settings: YMin=-0.04  YMax=0.09  SaveName=ScopeData14
  Actuators Dynamcis : Subsystem  TreatAsAtomicUnit=on
  Bus Creator : BusCreator  Inputs=12
  Bus Creator1 : BusCreator  Inputs=2
  Bus Selector : BusSelector  OutputSignals=Blockades,Blockade now,Reconfig signal
  Demux : Demux  Outputs=[13 6]
  Demux1 : Demux  Outputs=8
  F16 nlsim nlplant Asymetrical : MATLABFcn  MATLABFcn=nlplantASYM_Reconf  OutputDimensions=19  OutputSignalType=real
  Fidelity Flag : Constant  Value=fi_flag_Simulink
  Integrate F16 State Derivatives : Integrator  InitialCondition=trim_state
  Leading Edge Flap:Symetric deflection : Subsystem
  Model used flag : Constant  Value=Model_used_flag
  Mux1 : Mux  Inputs=8
  Mux2 : Mux  Inputs=[23 19]
  Mux5 : Mux  Inputs=[13 8 1 1]
  Rotation Angles to Direction Cosine Matrix : aerolibtransform2/Rotation Angles to Direction Cosine Matrix  rotationOrder=ZYX
  Selector : Selector  InputPortWidth=13  IndexOptions=Index vector (dialog)  Indices=[1:3]  OutputSizes=1
  Selector1 : Selector  InputPortWidth=13  IndexOptions=Index vector (dialog)  Indices=[1:3]  OutputSizes=1
  Selector2 : Selector  InputPortWidth=13  IndexOptions=Index vector (dialog)  Indices=[7]  OutputSizes=1
  Selector3 : Selector  InputPortWidth=13  IndexOptions=Index vector (dialog)  Indices=[8:9]  OutputSizes=1
  Selector4 : Selector  InputPortWidth=13  IndexOptions=Index vector (dialog)  Indices=[10:12]  OutputSizes=1
  Selector5 : Selector  InputPortWidth=13  IndexOptions=Index vector (dialog)  Indices=[4:6]  OutputSizes=1
  Selector6 : Selector  InputPortWidth=6  IndexOptions=Index vector (dialog)  Indices=[1:3]  OutputSizes=1
  Selector7 : Selector  InputPortWidth=3  IndexOptions=Index vector (dialog)  Indices=[3 2 1]  OutputSizes=1
  Selector9 : Selector  InputPortWidth=13  IndexOptions=Index vector (dialog)  Indices=[10:12]  OutputSizes=1
  Signal Specification : SignalSpecification  Dimensions=19
  Sum1 : Sum  Inputs=|++  SaturateOnIntegerOverflow=on  InputSameDT=on  OutDataTypeStr=Inherit: Same as first input
  Sum9 : Sum  Inputs=|++  SaturateOnIntegerOverflow=on  InputSameDT=on  OutDataTypeStr=Inherit: Same as first input
  Output_bus : Outport
  Actual control def : Outport  Port=2
  wires:
  Integrate F16 State Derivatives/1 -> Selector5/1, Selector4/1, Selector3/1, Selector2/1, Selector/1, Bus Creator/2  "States_out"
  Rotation Angles to Direction Cosine Matrix/1 -> Bus Creator/10  "DCM_b"
  Bus Creator/1 -> Output_bus/1, Leading Edge Flap:Symetric deflection/1(state)
  Fidelity Flag/1 -> Mux5/3
  Control Comands/1 -> Demux1/1
  States/1 -> Mux5/1
  Mux2/1 -> F16 nlsim nlplant Asymetrical/1  "INPUTS"
  F16 nlsim nlplant Asymetrical/1 -> Demux/1  "OUTPUTS"
  Actuators Dynamcis/2(Dec_Control_def) -> Mux5/2
  Model used flag/1 -> Mux5/4
  Demux1/8 -> Sum1/1
  Demux1/7 -> Sum9/1
  Leading Edge Flap:Symetric deflection/1(delta_lef (deg)) -> Bus Creator1/1, Sum1/2, Sum9/2  "Symetric_LEF_defl"
  Demux1/5 -> Mux1/5
  Demux1/3 -> Mux1/3
  Demux1/1 -> Mux1/1
  Demux1/2 -> Mux1/2
  Demux1/4 -> Mux1/4
  Demux1/6 -> Mux1/6
  Sum9/1 -> Mux1/7
  Sum1/1 -> Mux1/8
  Mux1/1 -> Actuators Dynamcis/1(Control_commands)
  Selector9/1 -> Acels actual/1
  Actuators Dynamcis/3(Throttle_meas) -> Bus Creator/12  "Throttle"
  Demux/1 -> Selector9/1, Bus Creator/1, Selector1/1, Integrate F16 State Derivatives/1  "States_dot_out"
  Selector/1 -> Bus Creator/4  "X_e"
  Selector1/1 -> Bus Creator/5  "V_e"
  Selector2/1 -> Bus Creator/6  "TAS"
  Selector3/1 -> Bus Creator/7  "alpha ; beta"
  Selector4/1 -> Bus Creator/8  "p;q;r"
  Selector5/1 -> Selector7/1, Bus Creator/9  "euler"
  Selector6/1 -> Bus Creator/11  "an_b_CG"
  Demux/2 -> Selector6/1, Bus Creator/3  "Other outs"
  Selector7/1 -> Rotation Angles to Direction Cosine Matrix/1
  Mux5/1 -> Mux2/1  "INPUTS"
  Signal Specification/1 -> Actuators Dynamcis/4(Reconfig signal), Mux2/2
  Reconf params/1 -> Bus Selector/1
  Bus Selector/3 -> Signal Specification/1  "<Reconfig signal>"
  Bus Selector/1 -> Actuators Dynamcis/2(Blockades)  "<Blockades>"
  Bus Selector/2 -> Actuators Dynamcis/3(Blockade now)  "<Blockade now>"
  Bus Creator1/1 -> Actual control def/1
  Actuators Dynamcis/1(Control Defl Plot) -> Bus Creator1/2  "actual_control_defl"

== system F16ASYM_Controlled_ACC/NDI/NDI: NO RECONFIG ==
  note: These two block MUST be evaluated at the same dynamics X
      | and control deflections delta*
      |
      |
      | delta* are a given set of control deflection: can be either the initial trim set
      | or the previous deflections
  Est reconf : Inport
  Angular_acc_des (rad/s^2) : Inport  Port=2
  All_meas : Inport  Port=3
  Control_defl for eval : Inport  Port=4
  Bus Selector : BusSelector  OutputSignals=signal1.omega_b meas (rad/s),signal2.q (Pa),signal1.Alt meas (m),signal1.V_TAS (m/s),signal1.AoA meas (rad),signal1.SS meas (rad),signal1.Throttle_meas
  Demux : Demux  Outputs=3
  Dim_less : Subsystem
  Inversion : Sum  Inputs=|+-
  Memory : Memory  X0=[0,0,0]
  Mom Coefficients gradient with control deflections at the given dynamics X: It performs perturbations theory arroun the given control deflections : MATLABFcn  MATLABFcn=Moms_Coeff_Grad_estimator  OutputDimensions=21  OutputSignalType=real
  Mux : Mux  Inputs=3
  Mux1 : Mux  Inputs=7
  Pre-Inverter : MATLAB Function  TreatAsAtomicUnit=on
  Reshape : Reshape  OutputDimensionality=Customize  OutputDimensions=[k_B,m_B]
  Terminator : Terminator
  Trim controls Asym In LEFs: Additionaly from dLEF : Constant  Commented=on  Value=[trim_control(1),trim_control(1),trim_control(2),-trim_control(2),trim_control(3),0,0]
  "f(x)  Mom Coefficients due to the dynamics: Coefficients model with control inputs " : MATLABFcn  MATLABFcn=Moms_Coeff_estimator  OutputDimensions=3  OutputSignalType=real
  Virtual Control Commands : Outport
  B online : Outport  Port=2
  Control_defl evald : Outport  Port=3
  Mom coef comm : Outport  Port=4
  wires:
  Est reconf/1 -> Terminator/1
  Reshape/1 -> B online/1
  Mom Coefficients gradient with control deflections at the given dynamics X: It performs perturbations theory arroun the given control deflections/1 -> Reshape/1
  Mux/1 -> Memory/1, Inversion/1
  Bus Selector/7 -> Mux1/6  "<Throttle_meas>"
  Mux1/1 -> Mom Coefficients gradient with control deflections at the given dynamics X: It performs perturbations theory arroun the given control deflections/1, "f(x)  Mom Coefficients due to the dynamics: Coefficients model with control inputs "/1
  Control_defl for eval/1 -> Mux1/7, Control_defl evald/1
  Bus Selector/6 -> Mux1/4  "<SS meas (rad)>"
  Bus Selector/5 -> Mux1/3  "<AoA meas (rad)>"
  Bus Selector/4 -> Mux1/2  "<V_TAS (m/s)>"
  Bus Selector/3 -> Mux1/1  "<Alt meas (m)>"
  "f(x)  Mom Coefficients due to the dynamics: Coefficients model with control inputs "/1 -> Inversion/2  "f(x) or C_x"
  Dim_less/3(C_N des) -> Mux/3
  Dim_less/2(C_M des) -> Mux/2
  Dim_less/1(C_L des) -> Mux/1
  Pre-Inverter/3(N_comm) -> Dim_less/3(N_comm)
  Pre-Inverter/2(M_comm) -> Dim_less/2(M_comm)
  Pre-Inverter/1(L_comm) -> Dim_less/1(L_comm)
  Bus Selector/2 -> Dim_less/4(q)  "<q (Pa)>"
  All_meas/1 -> Bus Selector/1
  Demux/1 -> Pre-Inverter/1(p_dot_comm)
  Demux/3 -> Pre-Inverter/3(r_dot_comm)
  Demux/2 -> Pre-Inverter/2(q_dot_comm)
  Angular_acc_des (rad/s^2)/1 -> Demux/1
  Bus Selector/1 -> Mux1/5, Pre-Inverter/4(omega_b)  "<omega_b meas (rad/s)>"
  Inversion/1 -> Virtual Control Commands/1
  Memory/1 -> Mom coef comm/1

== system F16ASYM_Controlled_ACC/NDI/NDI: RECONFIG ==
  note: These two block MUST be evaluated at the same dynamics X
      | and control deflections delta*
      |
      |
      | delta* are a given set of control deflection: can be either the initial trim set
      | or the previous deflections
  note: INPUTS
      | States:
      |
      | 1. Altitude
      | 2. TAS velocity
      | 3. alpha in rad
      | 4. beta in rads
      | 5. P
      | 6. Q
      | 7. R
      | 8. Throttle
      | 9. Elevator_L in deg
      | 10. Elevator_R in deg
      | 11. Aileron_L
      | 12. Aileron_R
      | 13. Rudder
      | 14. LEF_L
      | 15. LEF_R
      |
      | RECONFIGURATION PARAMETERS
      |
      | 16. mass  Estimated mass
      | 17. S_current_L
      | 18. S_current_R
      | 19. S_fin_current
      | 20. x_cg
      | 21. Jy
      | 22. Jxz
      | 23. Jz
      | 24. Jx
      | 25. EFF_el_L
      | 26. EFF_el_R
      | 27. EFF_ail_L
      | 28 EFF_ail_R
      | 29. EFF_rud
      | 30. EFF_lef_L
      | 31. EFF_lef_R
      | 32. Delta_C_Lift_X
      | 33. Delta_C_Drag_X
      | 34. Delta_C_m_X
  Est reconf : Inport
  Angular_acc_des (rad/s^2) : Inport  Port=2
  All_meas : Inport  Port=3
  Control_defl for eval : Inport  Port=4
  Bus Selector : BusSelector  OutputSignals=signal1.omega_b meas (rad/s),signal2.q (Pa),signal1.Alt meas (m),signal1.V_TAS (m/s),signal1.AoA meas (rad),signal1.SS meas (rad),signal1.Throttle_meas
  Bus Selector1 : BusSelector  OutputSignals=Reconfig signal
  Controls : Scope
      settings: SaveName=ScopeData19
  Demux : Demux  Outputs=3
  Dim_less : Subsystem
  Inversion : Sum  Inputs=|+-
  Memory : Memory  X0=[0,0,0]
  Mom Coefficients gradient with control deflections at the given dynamics X: It performs perturbations theory arroun the given control deflections : MATLABFcn  MATLABFcn=Moms_Coeff_Grad_Reconf_estimator  OutputDimensions=21  OutputSignalType=real
  Mux : Mux  Inputs=3
  Mux1 : Mux  Inputs=7
  Mux2 : Mux  Inputs=[15 19]
  Plant : Scope
      settings: SaveName=ScopeData11
  Pre-Inverter : MATLAB Function  TreatAsAtomicUnit=on
  Reshape : Reshape  OutputDimensionality=Customize  OutputDimensions=[k_B,m_B]
  Signal Specification : SignalSpecification  Dimensions=19
  Trim controls Asym In LEFs: Additionaly from dLEF : Constant  Commented=on  Value=[trim_control(1),trim_control(1),trim_control(2),-trim_control(2),trim_control(3),0,0]
  f(x)  Mom Coefficients due to the dynamics: Coefficients model with control inputs : MATLABFcn  MATLABFcn=Moms_Coeff_Reconf_estimator  OutputDimensions=3  OutputSignalType=real
  Virtual Control Commands : Outport
  B online : Outport  Port=2
  Control_defl evald : Outport  Port=3
  Mom coef comm : Outport  Port=4
  wires:
  Inversion/1 -> Controls/1, Virtual Control Commands/1
  Bus Selector/1 -> Pre-Inverter/4(omega_b), Mux1/5  "<omega_b meas (rad/s)>"
  Angular_acc_des (rad/s^2)/1 -> Demux/1
  Demux/2 -> Pre-Inverter/2(q_dot_comm)
  Demux/3 -> Pre-Inverter/3(r_dot_comm)
  Demux/1 -> Pre-Inverter/1(p_dot_comm)
  All_meas/1 -> Bus Selector/1
  Bus Selector/2 -> Dim_less/4(q)  "<q (Pa)>"
  Pre-Inverter/1(L_comm) -> Dim_less/1(L_comm)
  Pre-Inverter/2(M_comm) -> Dim_less/2(M_comm)
  Pre-Inverter/3(N_comm) -> Dim_less/3(N_comm)
  Dim_less/1(C_L des) -> Mux/1
  Dim_less/2(C_M des) -> Mux/2
  Dim_less/3(C_N des) -> Mux/3
  f(x)  Mom Coefficients due to the dynamics: Coefficients model with control inputs/1 -> Plant/1, Inversion/2  "f(x) or C_x"
  Bus Selector/3 -> Mux1/1  "<Alt meas (m)>"
  Bus Selector/4 -> Mux1/2  "<V_TAS (m/s)>"
  Bus Selector/5 -> Mux1/3  "<AoA meas (rad)>"
  Bus Selector/6 -> Mux1/4  "<SS meas (rad)>"
  Control_defl for eval/1 -> Mux1/7, Control_defl evald/1
  Bus Selector/7 -> Mux1/6  "<Throttle_meas>"
  Mux/1 -> Inversion/1, Memory/1
  Mom Coefficients gradient with control deflections at the given dynamics X: It performs perturbations theory arroun the given control deflections/1 -> Reshape/1
  Reshape/1 -> B online/1
  Est reconf/1 -> Bus Selector1/1
  Bus Selector1/1 -> Signal Specification/1  "<Reconfig signal>"
  Mux1/1 -> Mux2/1
  Mux2/1 -> Mom Coefficients gradient with control deflections at the given dynamics X: It performs perturbations theory arroun the given control deflections/1, f(x)  Mom Coefficients due to the dynamics: Coefficients model with control inputs/1
  Signal Specification/1 -> Mux2/2
  Memory/1 -> Mom coef comm/1

== system F16ASYM_Controlled_ACC/P controller + adaptive Crossed NN + AWU+Lim    in ACC /Body Rates Controller ==
  p_ref : Inport
  q_ref : Inport  Port=2
  r_ref : Inport  Port=3
  All_meas : Inport  Port=4
  Bus Creator : BusCreator
  Bus Creator1 : BusCreator
  Bus Creator2 : BusCreator
  Bus Selector : BusSelector  OutputSignals=signal1.omega_b meas (rad/s)
  Display1 : Display
  Mux : Mux  Inputs=3
  Ref Model and P Controller p : Adaptive_FaultTolerantControl/Ref Model and P Controller  tau=0.1  y_i=trim_state(10)  K_f=1  K_b=7
  Ref Model and P Controller q : Subsystem
  Ref Model and P Controller r : Adaptive_FaultTolerantControl/Ref Model and P Controller  tau=0.2  y_i=trim_state(12)  K_f=1  K_b=4
  Selector : Selector  InputPortWidth=3  IndexOptions=Index vector (dialog)  Indices=1  OutputSizes=1
  Selector1 : Selector  InputPortWidth=3  IndexOptions=Index vector (dialog)  Indices=2  OutputSizes=1
  Selector2 : Selector  InputPortWidth=3  IndexOptions=Index vector (dialog)  Indices=3  OutputSizes=1
  Sum : Sum  Inputs=+-|
  Sum1 : Sum  Inputs=+-|
  Sum2 : Sum  Inputs=+-|
  q_chanel vars : Outport
  p_chanel vars : Outport  Port=2
  r_chanel vars : Outport  Port=3
  Angular acc des (rad/s^2) : Outport  Port=4
  wires:
  All_meas/1 -> Bus Selector/1
  Bus Selector/1 -> Selector/1, Selector1/1, Selector2/1  "<omega_b meas (rad/s)>"
  p_ref/1 -> Ref Model and P Controller p/1
  Selector/1 -> Ref Model and P Controller p/2
  Ref Model and P Controller p/1 -> Mux/1
  Mux/1 -> Angular acc des (rad/s^2)/1
  q_ref/1 -> Ref Model and P Controller q/1(y_ref)
  Selector1/1 -> Ref Model and P Controller q/2(y_meas)
  r_ref/1 -> Ref Model and P Controller r/1
  Ref Model and P Controller q/1(y_des_dot) -> Mux/2
  Ref Model and P Controller r/1 -> Mux/3
  Ref Model and P Controller p/2 -> Bus Creator/1  "p_sf_dot"
  Ref Model and P Controller p/3 -> Sum/1, Bus Creator/2  "p_sf"
  Sum/1 -> Display1/1, Bus Creator/3  "p_err"
  Bus Creator/1 -> p_chanel vars/1
  Bus Creator1/1 -> q_chanel vars/1
  Bus Creator2/1 -> r_chanel vars/1
  Selector2/1 -> Ref Model and P Controller r/2
  Ref Model and P Controller p/4 -> Sum/2
  Ref Model and P Controller p/5 -> Bus Creator/4  "K_b_p"
  Ref Model and P Controller q/2(y_c_ff_dot) -> Bus Creator1/1  "q_sf_dot"
  Ref Model and P Controller q/3(y_c) -> Sum1/1, Bus Creator1/2  "q_sf"
  Sum1/1 -> Bus Creator1/3  "q_err"
  Ref Model and P Controller q/4(y_meas_out) -> Sum1/2
  Ref Model and P Controller q/5(k_b param) -> Bus Creator1/4  "K_b_q"
  Ref Model and P Controller r/2 -> Bus Creator2/1  "r_sf_dot"
  Ref Model and P Controller r/3 -> Sum2/1, Bus Creator2/2  "r_sf"
  Sum2/1 -> Bus Creator2/3  "r_err"
  Ref Model and P Controller r/4 -> Sum2/2
  Ref Model and P Controller r/5 -> Bus Creator2/4  "K_b_r"
